simulink model "Practica2"  (R2022a)
settings: Solver=ode4  StartTime=0.0  StopTime=100  FixedStep=0.001  RelTol=1e-3
settings Model: Creator=Anahi Monserrat  LastModifiedBy=Anahi Monserrat

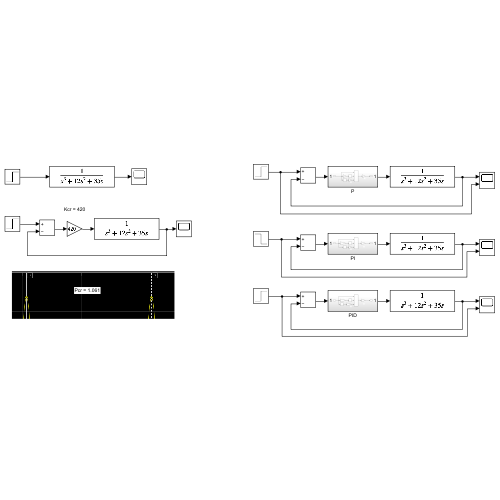
[thumbnail: Simulink's stored preview of the top-level diagram]
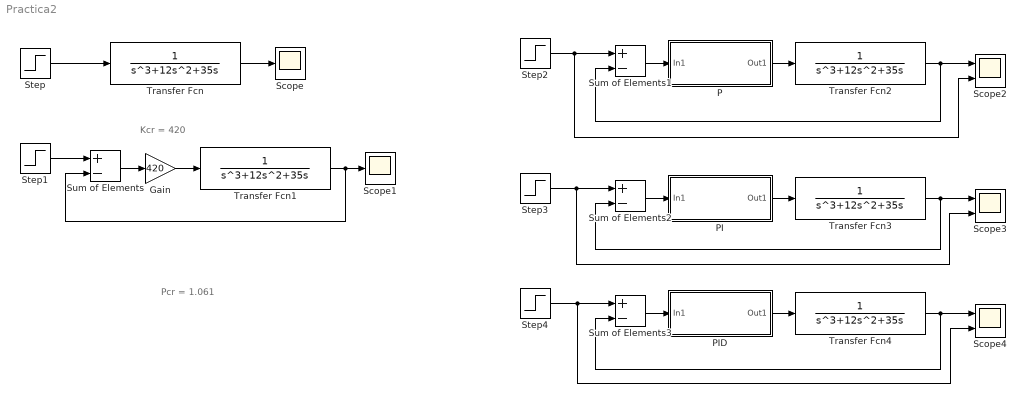
== system Practica2 ==
  note: Pcr = 1.061
  note: Kcr = 420
  Gain : Gain  Gain=420
  P : Subsystem
  PI : Subsystem
  PID : Subsystem
  Scope : Scope
  Scope1 : Scope
  Scope2 : Scope  NumInputPorts=2
  Scope3 : Scope  NumInputPorts=2
  Scope4 : Scope  NumInputPorts=2
  Step : Step  Time=0  SampleTime=0
  Step1 : Step  Time=0  SampleTime=0
  Step2 : Step  Time=10  SampleTime=0
  Step3 : Step  After=-5  SampleTime=0
  Step4 : Step  Time=0  SampleTime=0
  Sum of Elements{,1..3} (4 alike) : Sum  Inputs=+-
  Transfer Fcn{,1..4} (5 alike) : TransferFcn  Denominator=[1 12 35 0]
  wires:
  Step2/1 -> Scope2/2, Sum of Elements1/1
  Step3/1 -> Scope3/2, Sum of Elements2/1
  Transfer Fcn3/1 -> Sum of Elements2/2, Scope3/1
  Sum of Elements/1 -> Gain/1
  PI/1(Out1) -> Transfer Fcn3/1
  Gain/1 -> Transfer Fcn1/1
  Transfer Fcn2/1 -> Scope2/1, Sum of Elements1/2
  P/1(Out1) -> Transfer Fcn2/1
  PID/1(Out1) -> Transfer Fcn4/1
  Sum of Elements3/1 -> PID/1(In1)
  Step4/1 -> Scope4/2, Sum of Elements3/1
  Sum of Elements2/1 -> PI/1(In1)
  Transfer Fcn4/1 -> Scope4/1, Sum of Elements3/2
  Transfer Fcn1/1 -> Sum of Elements/2, Scope1/1
  Step1/1 -> Sum of Elements/1
  Sum of Elements1/1 -> P/1(In1)
  Step/1 -> Transfer Fcn/1
  Transfer Fcn/1 -> Scope/1

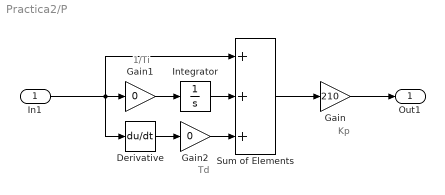
== system Practica2/P ==
  note: Kp
  note: Td
  note: 1/Ti
  In1 : Inport
  Derivative : Derivative
  Gain : Gain  Gain=210
  Gain1 : Gain  Gain=0
  Gain2 : Gain  Gain=0
  Integrator : Integrator
  Sum of Elements : Sum  Inputs=+++
  Out1 : Outport
  wires:
  Sum of Elements/1 -> Gain/1
  In1/1 -> Derivative/1, Sum of Elements/1, Gain1/1
  Integrator/1 -> Sum of Elements/2
  Gain1/1 -> Integrator/1
  Gain/1 -> Out1/1
  Derivative/1 -> Gain2/1
  Gain2/1 -> Sum of Elements/3

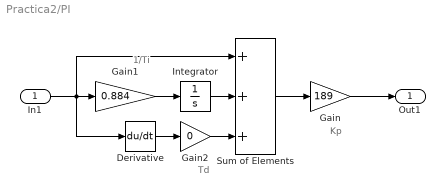
== system Practica2/PI ==
  note: Kp
  note: 1/Ti
  note: Td
  In1 : Inport
  Derivative : Derivative
  Gain : Gain  Gain=189
  Gain1 : Gain  Gain=0.884
  Gain2 : Gain  Gain=0
  Integrator : Integrator
  Sum of Elements : Sum  Inputs=+++
  Out1 : Outport
  wires:
  Gain2/1 -> Sum of Elements/3
  Derivative/1 -> Gain2/1
  Gain/1 -> Out1/1
  Gain1/1 -> Integrator/1
  Integrator/1 -> Sum of Elements/2
  Sum of Elements/1 -> Gain/1
  In1/1 -> Sum of Elements/1, Derivative/1, Gain1/1

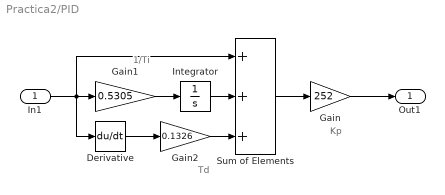
== system Practica2/PID ==
  note: Td
  note: 1/Ti
  note: Kp
  In1 : Inport
  Derivative : Derivative
  Gain : Gain  Gain=252
  Gain1 : Gain  Gain=0.5305
  Gain2 : Gain  Gain=0.1326
  Integrator : Integrator
  Sum of Elements : Sum  Inputs=+++
  Out1 : Outport
  wires:
  In1/1 -> Gain1/1, Derivative/1, Sum of Elements/1
  Sum of Elements/1 -> Gain/1
  Integrator/1 -> Sum of Elements/2
  Gain1/1 -> Integrator/1
  Gain/1 -> Out1/1
  Derivative/1 -> Gain2/1
  Gain2/1 -> Sum of Elements/3
